simulink model "ResampleFL3Model"  (Simulink 6.6)
settings: Solver=FixedStepDiscrete  StartTime=0.0  StopTime=0  FixedStep=0.1  RelTol=1e-3
libraries: SimITKLibraryFL3 x4, SimITKTransformLibrary3D x1
settings Model: Creator=3kml  LastModifiedBy=3kml

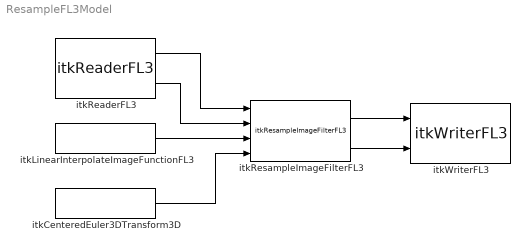
== system ResampleFL3Model ==
  itkCenteredEuler3DTransform3D : SimITKTransformLibrary3D/itkCenteredEuler3DTransform3D  Parameters_a=[0 0 20 127.5 127.5 90 0 0 0]  FixedParameters=[]
  itkLinearInterpolateImageFunctionFL3 : SimITKLibraryFL3/itkLinearInterpolateImageFunctionFL3
  itkReaderFL3 : SimITKLibraryFL3/itkReaderFL3  FileName='subject04_t1w_p4_float.mha'
  itkResampleImageFilterFL3 : SimITKLibraryFL3/itkResampleImageFilterFL3  DefaultPixelValue=0  OutputOrigin=[0 0 0]  OutputSpacing=[1 1 1]  Size=[256 256 181]
  itkWriterFL3 : SimITKLibraryFL3/itkWriterFL3  FileName='outputResampleFL3Model.mhd'
  wires:
  itkResampleImageFilterFL3/1 -> itkWriterFL3/1
  itkResampleImageFilterFL3/2 -> itkWriterFL3/2
  itkReaderFL3/1 -> itkResampleImageFilterFL3/1
  itkReaderFL3/2 -> itkResampleImageFilterFL3/2
  itkLinearInterpolateImageFunctionFL3/1 -> itkResampleImageFilterFL3/3
  itkCenteredEuler3DTransform3D/1 -> itkResampleImageFilterFL3/4
